simulink model "slider_crank"  (R2024b)
settings: Solver=VariableStepAuto  StartTime=0.0  StopTime=10.0  RelTol=1e-3
settings Model: Creator=henry  LastModifiedBy=henry

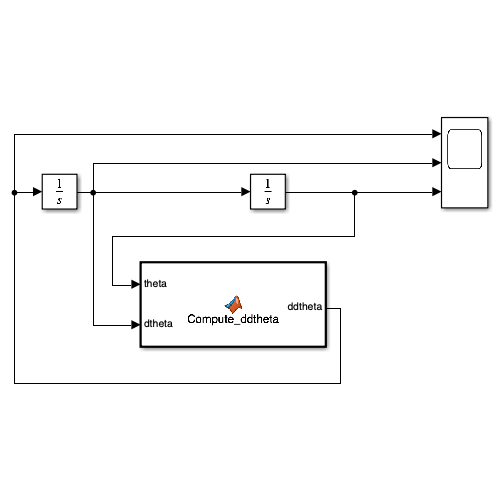
[thumbnail: Simulink's stored preview of the top-level diagram]
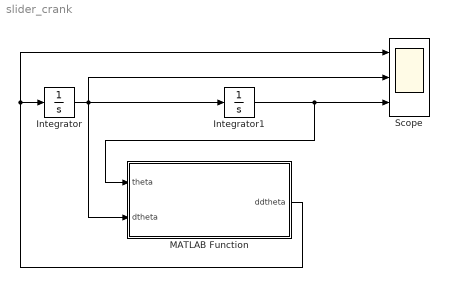
== system slider_crank ==
  Integrator : Integrator  InitialCondition=10
  Integrator1 : Integrator  InitialCondition=1.05
  MATLAB Function : MATLAB Function  TreatAsAtomicUnit=on
  Scope : Scope  NumInputPorts=3
  wires:
  Integrator/1 -> Scope/2, MATLAB Function/2(dtheta), Integrator1/1
  Integrator1/1 -> MATLAB Function/1(theta), Scope/3
  MATLAB Function/1(ddtheta) -> Scope/1, Integrator/1

== matlab function slider_crank/MATLAB Function ==
  data: theta input; ddtheta output; dtheta input
function ddtheta = Compute_ddtheta(theta, dtheta)
%#codegen

% 参数（可以在工作区设置）
m1 = 1.0; m2 = 2.0; m3 = 0.5;
l1 = 0.3; l2 = 0.5; g = 9.81;

[M, dM] = massFunction(theta, m1, m2, m3, l1, l2);

ddtheta = - (0.5*dM*dtheta^2 + 0.5*(m1 + m2)*g*l1*cos(theta)) / M;
